simulink model "PID_validation_2_2_2"  (R2024b)
settings: Solver=FixedStepAuto  StartTime=0.0  StopTime=40  FixedStep=0.0001  RelTol=1e-3
undefined symbols (not defined in the file): daq, drv, gbox, K_W, kd, ki, kp, mld, mot, rads2rpm, sens, step_gain, tl, Ts, u_bar_max
settings Model: Creator=Enrico  LastModifiedBy=Enrico 2
settings DataIOCC: ReturnWorkspaceOutputsName=out_black_box

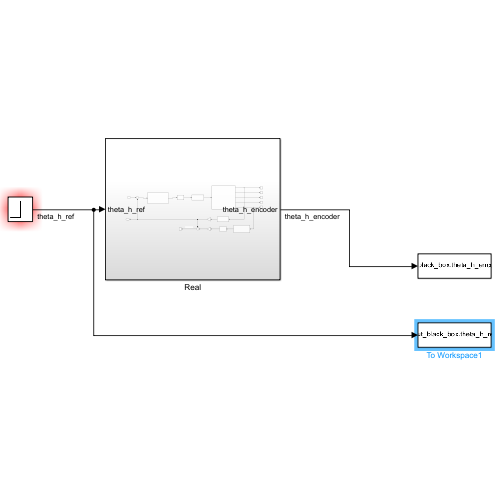
[thumbnail: Simulink's stored preview of the top-level diagram]
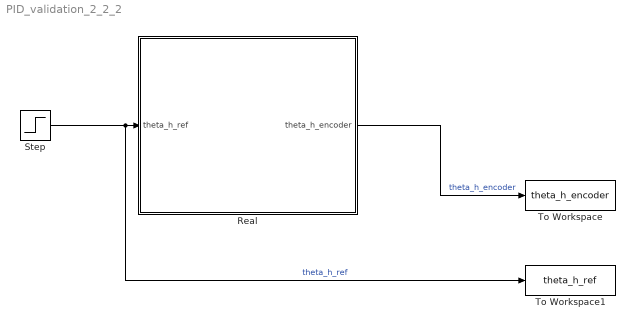
== system PID_validation_2_2_2 ==
  Real : Subsystem
  Step : Step  After=step_gain  SampleTime=0
  To Workspace : ToWorkspace  VariableName=theta_h_encoder  SaveFormat=Structure With Time  SampleTime=-1
  To Workspace1 : ToWorkspace  VariableName=theta_h_ref  SaveFormat=Structure With Time  SampleTime=-1
  wires:
  Step/1 -> To Workspace1/1, Real/1(theta_h_ref)  "theta_h_ref"
  Real/1(theta_h_encoder) -> To Workspace/1  "theta_h_encoder"

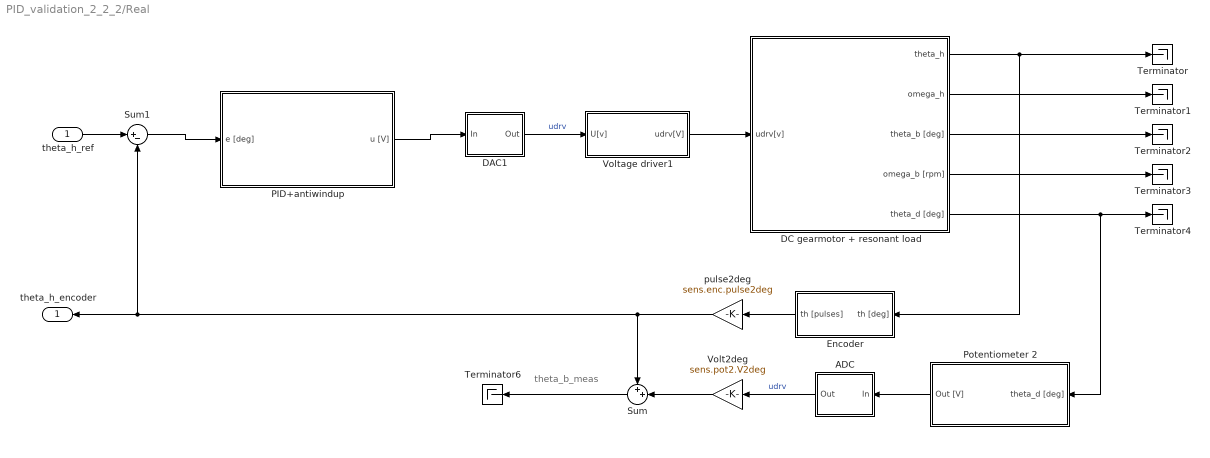
== system PID_validation_2_2_2/Real ==
  note: theta_b_meas
  theta_h_ref : Inport
  ADC : Subsystem
  DAC1 : Subsystem
  DC gearmotor + resonant load : Subsystem
  Encoder : Subsystem
  PID+antiwindup : Subsystem
  Potentiometer 2 : Subsystem
  Sum : Sum  Inputs=++|
  Sum1 : Sum  Inputs=|+-
  Terminator{,1..4,6} (6 alike) : Terminator
  Volt2deg : Gain  Gain=sens.pot2.V2deg
  Voltage driver1 : Subsystem
  pulse2deg : Gain  Gain=sens.enc.pulse2deg
  theta_h_encoder : Outport
  wires:
  DC gearmotor + resonant load/1(theta_h) -> Terminator/1, Encoder/1(th [deg])
  pulse2deg/1 -> Sum1/2, theta_h_encoder/1, Sum/1
  Sum/1 -> Terminator6/1
  DC gearmotor + resonant load/5(theta_d [deg]) -> Potentiometer 2/1(theta_d [deg]), Terminator4/1
  PID+antiwindup/1(u [V]) -> DAC1/1(In)
  DC gearmotor + resonant load/4(omega_b [rpm]) -> Terminator3/1
  Voltage driver1/1(udrv[V]) -> DC gearmotor + resonant load/1(udrv[v])
  Encoder/1(th [pulses]) -> pulse2deg/1
  theta_h_ref/1 -> Sum1/1
  DAC1/1(Out) -> Voltage driver1/1(U[v])  "udrv"
  DC gearmotor + resonant load/2(omega_h) -> Terminator1/1
  DC gearmotor + resonant load/3(theta_b [deg]) -> Terminator2/1
  Volt2deg/1 -> Sum/2
  Potentiometer 2/1(Out [V]) -> ADC/1(In)
  Sum1/1 -> PID+antiwindup/1(e [deg])
  ADC/1(Out) -> Volt2deg/1  "udrv"

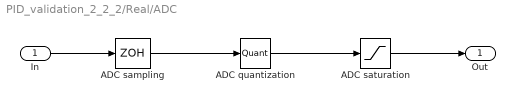
== system PID_validation_2_2_2/Real/ADC ==
  In : Inport
  ADC quantization : Quantizer  QuantizationInterval=daq.adc.q
  ADC sampling : ZeroOrderHold  SampleTime=Ts
  ADC saturation : Saturate  UpperLimit=daq.adc.fs  LowerLimit=-daq.adc.fs
  Out : Outport
  wires:
  ADC quantization/1 -> ADC saturation/1
  In/1 -> ADC sampling/1
  ADC sampling/1 -> ADC quantization/1
  ADC saturation/1 -> Out/1

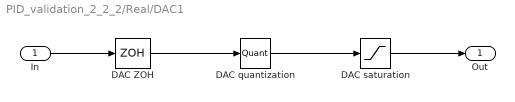
== system PID_validation_2_2_2/Real/DAC1 ==
  In : Inport
  DAC ZOH : ZeroOrderHold  SampleTime=Ts
  DAC quantization : Quantizer  QuantizationInterval=daq.dac.q
  DAC saturation : Saturate  UpperLimit=daq.dac.fs  LowerLimit=-daq.dac.fs
  Out : Outport
  wires:
  DAC quantization/1 -> DAC saturation/1
  In/1 -> DAC ZOH/1
  DAC ZOH/1 -> DAC quantization/1
  DAC saturation/1 -> Out/1

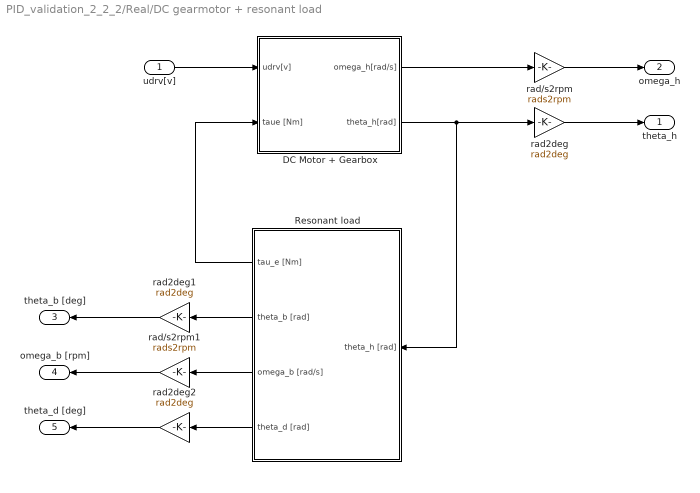
== system PID_validation_2_2_2/Real/DC gearmotor + resonant load ==
  udrv[v] : Inport
  DC Motor + Gearbox : Subsystem
  Resonant load : Subsystem
  rad/s2rpm : Gain  Gain=rads2rpm
  rad/s2rpm1 : Gain  Gain=rads2rpm
  rad2deg : Gain  Gain=rad2deg
  rad2deg1 : Gain  Gain=rad2deg
  rad2deg2 : Gain  Gain=rad2deg
  theta_h : Outport
  omega_h : Outport  Port=2
  theta_b [deg] : Outport  Port=3
  omega_b [rpm] : Outport  Port=4
  theta_d [deg] : Outport  Port=5
  wires:
  udrv[v]/1 -> DC Motor + Gearbox/1(udrv[v])
  DC Motor + Gearbox/2(theta_h[rad]) -> rad2deg/1, Resonant load/1(theta_h [rad])
  Resonant load/3(omega_b [rad/s]) -> rad/s2rpm1/1
  Resonant load/2(theta_b [rad]) -> rad2deg1/1
  Resonant load/1(tau_e [Nm]) -> DC Motor + Gearbox/2(taue [Nm])
  rad/s2rpm1/1 -> omega_b [rpm]/1
  rad2deg2/1 -> theta_d [deg]/1
  rad2deg1/1 -> theta_b [deg]/1
  Resonant load/4(theta_d [rad]) -> rad2deg2/1
  rad/s2rpm/1 -> omega_h/1
  DC Motor + Gearbox/1(omega_h[rad/s]) -> rad/s2rpm/1
  rad2deg/1 -> theta_h/1

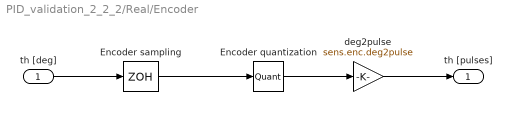
== system PID_validation_2_2_2/Real/Encoder ==
  th [deg] : Inport
  Encoder quantization : Quantizer  QuantizationInterval=sens.enc.pulse2deg
  Encoder sampling : ZeroOrderHold  SampleTime=Ts
  deg2pulse : Gain  Gain=sens.enc.deg2pulse
  th [pulses] : Outport
  wires:
  Encoder quantization/1 -> deg2pulse/1
  th [deg]/1 -> Encoder sampling/1
  Encoder sampling/1 -> Encoder quantization/1
  deg2pulse/1 -> th [pulses]/1

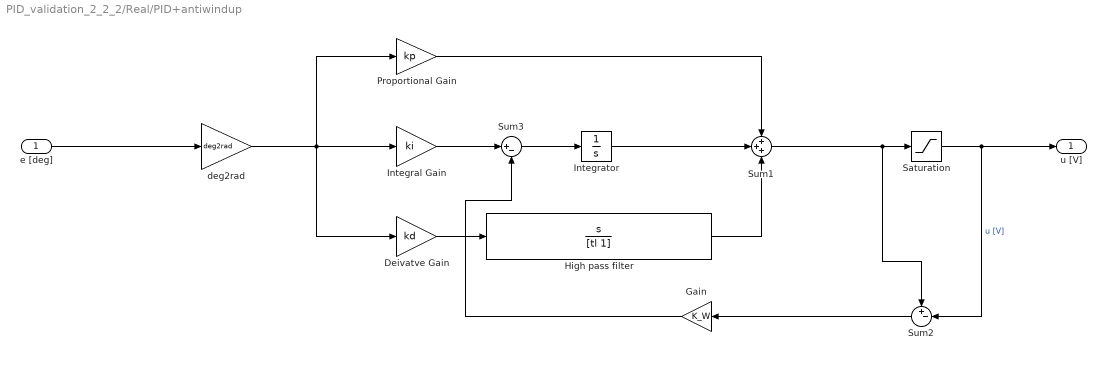
== system PID_validation_2_2_2/Real/PID+antiwindup ==
  e [deg] : Inport
  Deivatve Gain : Gain  Gain=kd
  Gain : Gain  Gain=K_W
  High pass filter : TransferFcn  Numerator=[1 0]  Denominator=[tl 1]
  Integral Gain : Gain  Gain=ki
  Integrator : Integrator
  Proportional Gain : Gain  Gain=kp
  "Saturation " : Saturate  UpperLimit=u_bar_max  LowerLimit=-u_bar_max
  Sum1 : Sum  Inputs=+++
  Sum2 : Sum  Inputs=+-|
  Sum3 : Sum  Inputs=|+-
  deg2rad : Gain  Gain=deg2rad
  u [V] : Outport
  wires:
  Integrator/1 -> Sum1/2
  e [deg]/1 -> deg2rad/1
  Sum3/1 -> Integrator/1
  Sum1/1 -> Sum2/1, "Saturation "/1
  Sum2/1 -> Gain/1
  Proportional Gain/1 -> Sum1/1
  deg2rad/1 -> Deivatve Gain/1, Proportional Gain/1, Integral Gain/1
  High pass filter/1 -> Sum1/3
  Integral Gain/1 -> Sum3/1
  "Saturation "/1 -> Sum2/2, u [V]/1  "u [V]"
  Deivatve Gain/1 -> High pass filter/1
  Gain/1 -> Sum3/2

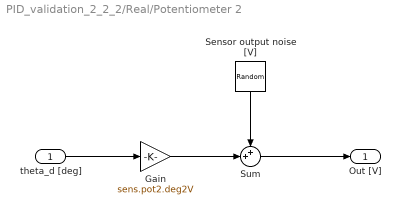
== system PID_validation_2_2_2/Real/Potentiometer 2 ==
  theta_d [deg] : Inport
  Gain : Gain  Gain=sens.pot2.deg2V
  Sensor output noise [V] : RandomNumber  SampleTime=Ts
  Sum : Sum  Inputs=++|
  Out [V] : Outport
  wires:
  theta_d [deg]/1 -> Gain/1
  Sum/1 -> Out [V]/1
  Gain/1 -> Sum/2
  Sensor output noise [V]/1 -> Sum/1

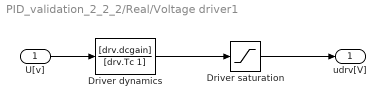
== system PID_validation_2_2_2/Real/Voltage driver1 ==
  U[v] : Inport
  Driver dynamics : TransferFcn  Numerator=[drv.dcgain]  Denominator=[drv.Tc 1]
  Driver saturation : Saturate  UpperLimit=12  LowerLimit=-12
  udrv[V] : Outport
  wires:
  U[v]/1 -> Driver dynamics/1
  Driver dynamics/1 -> Driver saturation/1
  Driver saturation/1 -> udrv[V]/1

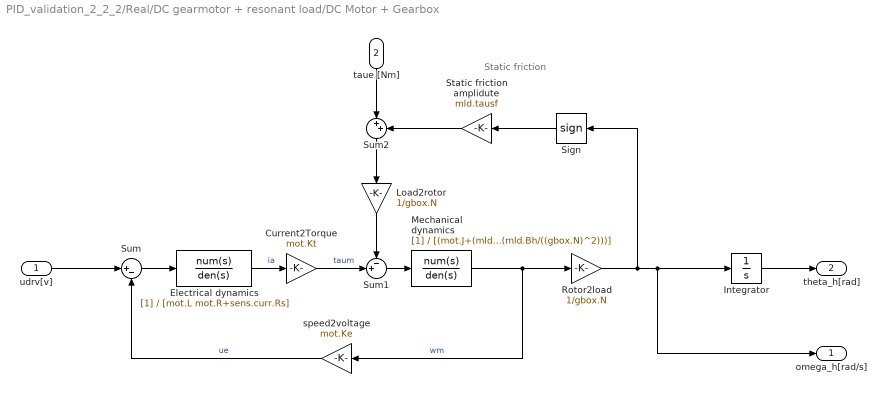
== system PID_validation_2_2_2/Real/DC gearmotor + resonant load/DC Motor + Gearbox ==
  note: Static friction
  udrv[v] : Inport
  taue [Nm] : Inport  Port=2
  " Sign" : Signum  ZeroCross=off
  Current2Torque : Gain  Gain=mot.Kt
  Electrical dynamics : TransferFcn  Denominator=[mot.L mot.R+sens.curr.Rs]
  Integrator : Integrator
  Load2rotor : Gain  Gain=1/gbox.N
  Mechanical dynamics : TransferFcn  Denominator=[(mot.J+(mld.Jh/((gbox.N)^2))) (mot.B+(mld.Bh/((gbox.N)^2)))]
  Rotor2load : Gain  Gain=1/gbox.N
  Static friction amplidute : Gain  Gain=mld.tausf
  Sum : Sum  Inputs=|+-
  Sum1 : Sum  Inputs=-+|
  Sum2 : Sum  Inputs=|++
  speed2voltage : Gain  Gain=mot.Ke
  omega_h[rad/s] : Outport
  theta_h[rad] : Outport  Port=2
  wires:
  udrv[v]/1 -> Sum/1
  Sum/1 -> Electrical dynamics/1
  Electrical dynamics/1 -> Current2Torque/1  "ia"
  Current2Torque/1 -> Sum1/2  "taum"
  Load2rotor/1 -> Sum1/1
  " Sign"/1 -> Static friction amplidute/1
  Sum1/1 -> Mechanical dynamics/1
  Mechanical dynamics/1 -> speed2voltage/1, Rotor2load/1  "wm"
  speed2voltage/1 -> Sum/2  "ue"
  Rotor2load/1 -> " Sign"/1, omega_h[rad/s]/1, Integrator/1
  Sum2/1 -> Load2rotor/1
  Static friction amplidute/1 -> Sum2/2
  taue [Nm]/1 -> Sum2/1
  Integrator/1 -> theta_h[rad]/1

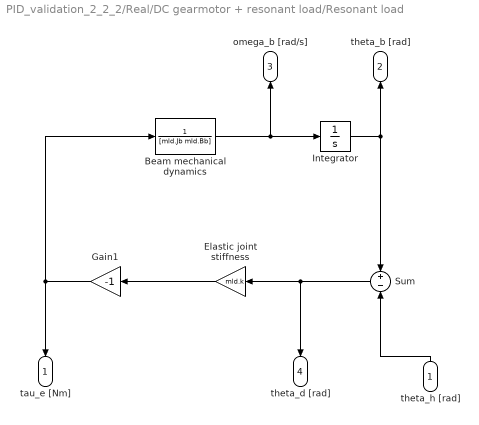
== system PID_validation_2_2_2/Real/DC gearmotor + resonant load/Resonant load ==
  theta_h [rad] : Inport
  Beam mechanical dynamics : TransferFcn  Denominator=[mld.Jb mld.Bb]
  Elastic joint stiffness : Gain  Gain=mld.k
  Gain1 : Gain  Gain=-1
  Integrator : Integrator
  Sum : Sum  Inputs=+|-
  tau_e [Nm] : Outport
  theta_b [rad] : Outport  Port=2
  omega_b [rad/s] : Outport  Port=3
  theta_d [rad] : Outport  Port=4
  wires:
  theta_h [rad]/1 -> Sum/2
  Gain1/1 -> tau_e [Nm]/1, Beam mechanical dynamics/1
  Sum/1 -> Elastic joint stiffness/1, theta_d [rad]/1
  Integrator/1 -> theta_b [rad]/1, Sum/1
  Elastic joint stiffness/1 -> Gain1/1
  Beam mechanical dynamics/1 -> omega_b [rad/s]/1, Integrator/1
